simulink model "rvs_prototypes"  (R2016a)
settings: Solver=ode45  StartTime=0.0  StopTime=10.0  RelTol=1e-3
libraries: simulink x2
settings Model: Creator=Arthur  LastModifiedBy=aeagr
settings DataIOCC: LimitDataPoints=on  SaveFormat=Array
settings DebuggingCC: SolverPrmCheckMsg=warning
settings HardwareCC: ProdBitPerPointer=32  ProdLargestAtomicFloat=None  ProdIntDivRoundTo=Undefined  ProdEndianess=Unspecified  ProdWordSize=32  ProdHWDeviceType=32-bit Generic
settings ModelReferenceCC: PropagateSignalLabelsOutOfModel=off
settings ConfigComp: CovModelRefEnable=Off  CovSFcnEnable=off

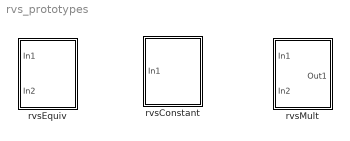
== system rvs_prototypes ==
  rvsConstant : Subsystem  TreatAsAtomicUnit=on  mask(rvsConstant){}
      mask help: Require that the input signal must be constant
  rvsEquiv : Subsystem  TreatAsAtomicUnit=on  mask(rvsEquiv){tol=1e-9}
      mask prompts: tol "Equality tolerance"
      mask help: Test equivalence between two input signals.
  rvsMult : Subsystem  TreatAsAtomicUnit=on  mask(rvsMult){}
      mask help: Matrix multiplication of two input signals.

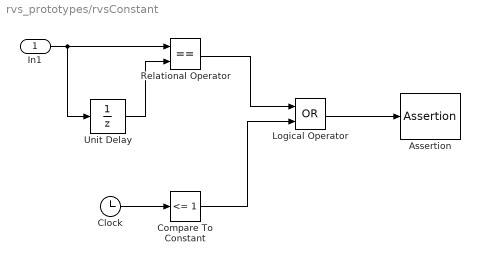
== system rvs_prototypes/rvsConstant ==
  In1 : Inport
  Assertion : Assertion
  Clock : Clock
  Compare To Constant : simulink/Logic and Bit Operations/Compare To Constant  relop=<=  const=1  OutDataTypeStr=boolean
  Logical Operator : Logic  Operator=OR  AllPortsSameDT=off  OutDataTypeStr=boolean
  Relational Operator : RelationalOperator  Operator===  OutDataTypeStr=boolean
  Unit Delay : UnitDelay  SampleTime=-1
  wires:
  In1/1 -> Unit Delay/1, Relational Operator/1
  Unit Delay/1 -> Relational Operator/2
  Logical Operator/1 -> Assertion/1
  Relational Operator/1 -> Logical Operator/1
  Clock/1 -> Compare To Constant/1
  Compare To Constant/1 -> Logical Operator/2

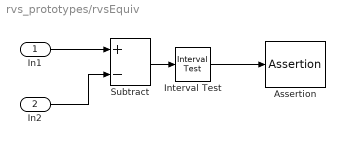
== system rvs_prototypes/rvsEquiv ==
  In1 : Inport
  In2 : Inport  Port=2
  Assertion : Assertion
  Interval Test : simulink/Logic and Bit Operations/Interval Test  IntervalClosedRight=on  uplimit=tol  IntervalClosedLeft=on  lowlimit=-tol  OutDataTypeStr=boolean
  Subtract : Sum  Inputs=+-
  wires:
  Interval Test/1 -> Assertion/1
  In2/1 -> Subtract/2
  In1/1 -> Subtract/1
  Subtract/1 -> Interval Test/1

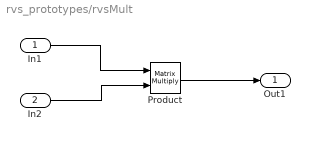
== system rvs_prototypes/rvsMult ==
  In1 : Inport
  In2 : Inport  Port=2
  Product : Product  Multiplication=Matrix(*)
  Out1 : Outport
  wires:
  In1/1 -> Product/1
  In2/1 -> Product/2
  Product/1 -> Out1/1
